simulink model "L7"  (R2023b)
settings: Solver=VariableStepAuto  StartTime=0.0  StopTime=100  MaxStep=0.01  RelTol=1e-3
values from neighbouring files (symbols this model uses):
  Ad = [ 0 1 0 ; 0 0 1 ;  -m0  -m1  -m2 ]    [mL7.m]
  Bd = [ 0 ; 0 ; 1 ]    [mL7.m]
  Cd = [ n0   n1   n2 ]    [mL7.m]
  F = acker (Ad,Bd,poles_mr)    [mL7.m]
  K = 1/pmr_ust    [mL7.m]
  K1 = 0.5    [mL7.m]
  K2 = 0.1    [mL7.m]
  Kg = 1/(K1*K2)    (= 20)    [mL7.m]
  m0 = Wzoh_plant.Denominator{1}(4)    [mL7.m]
  m1 = Wzoh_plant.Denominator{1}(3)    [mL7.m]
  m2 = Wzoh_plant.Denominator{1}(2)    [mL7.m]
  q = 0.2    [mL7.m]
  T1 = 4    [mL7.m]
  T2 = 5    [mL7.m]
  T3 = 1    [mL7.m]
  Ts = 0.1* (T1 + T2 + T3)    (= 1)    [mL7.m]
  Un = 80    [mL7.m]
settings Model: Creator=td  LastModifiedBy=killer
settings SolverCC: AlgebraicLoopSolver=TrustRegion
settings DataIOCC: ReturnWorkspaceOutputs=off
settings DebuggingCC: UnconnectedInputMsg=warning  UnconnectedOutputMsg=warning  UnconnectedLineMsg=warning  ArithmeticOperatorsInVariantConditions=warning
settings ModelReferenceCC: EnableRefExpFcnMdlSchedulingChecks=on
settings SFSimCC: CustomCodeUndefinedFunction=UseInterfaceOnly

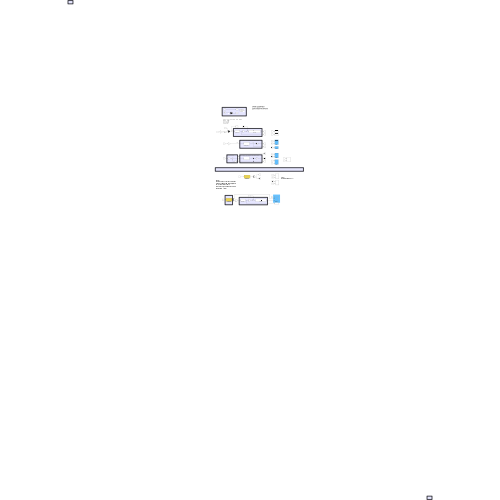
[thumbnail: Simulink's stored preview of the top-level diagram]
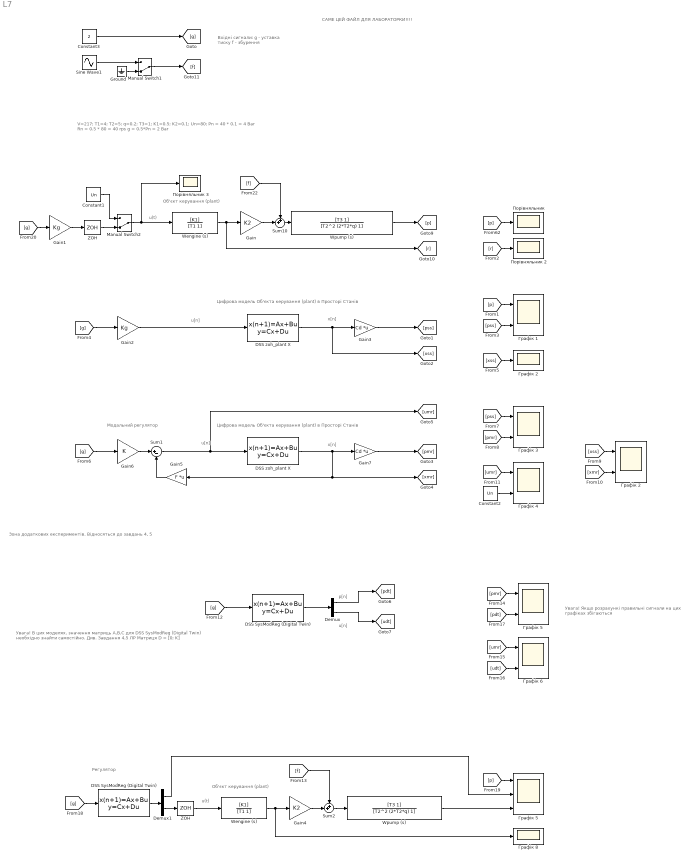
== system L7 ==
  note: Увага!
      | В цих моделях, значення матриць A,B,C для DSS SysModReg (Digital Twin) необхідно знайти самостійно. Див. Завдання 4,5 ЛР
      | Матриця D = [0; K]
  note: Зона додаткових експериментів. Відносяться до завдань 4, 5
  note: Регулятор
  note: Модальний регулятор
  note: x[n]
  note: u(t)
  note: V=217; T1=4; T2=5; q=0.2; T3=1; K1=0.5; K2=0.1; Un=80;
      |
      | Pn = 40 * 0.1 = 4 Bar
      | Rn = 0.5 * 80 = 40 rps
      |
      | g = 0.5*Pn = 2 Bar
  note: Вхідні сигнали:
      |
      | g - уставка тиску
      |
      | f - збурення
  note: САМЕ ЦЕЙ ФАЙЛ
      | ДЛЯ ЛАБОРАТОРКИ!!!!
  note: Об'єкт керування (plant)
  note: Цифрова модель Об'єкта керування (plant) в Просторі Станів
  note: u[n]
  note: Цифрова модель Об'єкта керування (plant) в Просторі Станів
  note: u[n]
  note: x[n]
  note: u(t)
  note: Об'єкт керування (plant)
  note: u[n]
  note: p[n]
  note: Увага!
      | Якщо розрахункі правильні
      | сигнали на цих графіках збігаються
  "  Wpump (s)" : TransferFcn  Numerator=[T3 1]  Denominator=[T2^2 (2*T2*q) 1]
  "  Wpump (s) " : TransferFcn  Numerator=[T3 1]  Denominator=[T2^2 (2*T2*q) 1]
  " DSS SysModReg (Digital Twin)" : DiscreteStateSpace  A=(Ad-Bd*F)  B=Bd*K  C=[Cd; -F]  D=[0; K]  SampleTime=Ts
  " DSS SysModReg (Digital Twin) " : DiscreteStateSpace  A=Ad-Bd*F  B=Bd*K  C=[Cd; -F]  D=[0; K]  SampleTime=Ts
  " DSS zoh_plant X" : DiscreteStateSpace  A="[ 0 1 0 ; 0 0 1 ;  -m0  -m1  -m2 ]"  B=[ 0 ; 0 ; 1 ]  C=eye(3)  D=[0;0;0]  SampleTime=Ts
  " DSS zoh_plant X " : DiscreteStateSpace  A="[ 0 1 0 ; 0 0 1 ;  -m0  -m1  -m2 ]"  B=[ 0 ; 0 ; 1 ]  C=[1 0 0; 0 1 0; 0 0 1]  D=[0;0;0]  SampleTime=Ts
  " ZOH " : ZeroOrderHold  SampleTime=Ts
  " Графік 2" : Scope
  " Графік 5  " : Scope  NumInputPorts=3
  " Порівняльник " : Scope
  " Порівняльник 2" : Scope
  " Порівняльник 3" : Scope
  Constant1 : Constant  Value=Un
  Constant2 : Constant  Value=Un
  Constant3 : Constant  Value=2
  Demux : Demux  Outputs=2
  Demux1 : Demux  Outputs=2
  Gain : Gain  Gain=K2
  Gain1 : Gain  Gain=Kg
  Gain2 : Gain  Gain=Kg
  Gain3 : Gain  Gain=Cd  Multiplication=Matrix(K*u)
  Gain4 : Gain  Gain=K2
  Gain5 : Gain  Gain=F  Multiplication=Matrix(K*u)
  Gain6 : Gain  Gain=K
  Gain7 : Gain  Gain=Cd  Multiplication=Matrix(K*u)
  Ground : Ground
  Manual Switch1 : ManualSwitch  CurrentSetting=0
  Manual Switch2 : ManualSwitch  CurrentSetting=0
  Sine Wave1 : Sin  Amplitude=5  Frequency=0.4  SampleTime=Ts
  Sum1 : Sum  Inputs=|+-
  Sum10 : Sum  Inputs=++|
  Sum2 : Sum  Inputs=++|
  "Wengine (s) " : TransferFcn  Numerator=[K1]  Denominator=[T1 1]
  "Wengine (s)  " : TransferFcn  Numerator=[K1]  Denominator=[T1 1]
  ZOH : ZeroOrderHold  SampleTime=Ts
  Графік {1..6} (6 alike) : Scope  NumInputPorts=2
  Графік 8 : Scope
  wires:
  Sine Wave1/1 -> Manual Switch1/1
  Gain/1 -> Sum10/2
  Sum10/1 -> "  Wpump (s)"/1
  Manual Switch1/1 -> [f]
  "  Wpump (s)"/1 -> [p]
  [f] -> Sum10/1
  Constant3/1 -> [g]
  "Wengine (s) "/1 -> Gain/1, [r]
  [p] -> " Порівняльник "/1
  Manual Switch2/1 -> "Wengine (s) "/1, " Порівняльник 3"/1
  ZOH/1 -> Manual Switch2/2
  Constant1/1 -> Manual Switch2/1
  Ground/1 -> Manual Switch1/2
  [r] -> " Порівняльник 2"/1
  Gain1/1 -> ZOH/1
  [g] -> Gain1/1
  Gain2/1 -> " DSS zoh_plant X "/1
  " DSS zoh_plant X "/1 -> [xss], Gain3/1
  Gain3/1 -> [pss]
  [p] -> Графік 1/1
  [pss] -> Графік 1/2
  [g] -> Gain2/1
  [xss] -> " Графік 2"/1
  " DSS zoh_plant X"/1 -> Gain5/1, [xmr], Gain7/1
  Gain7/1 -> [pmr]
  [g] -> Gain6/1
  Gain6/1 -> Sum1/1
  Sum1/1 -> [umr], " DSS zoh_plant X"/1
  Gain5/1 -> Sum1/2
  [pmr] -> Графік 3/2
  [pss] -> Графік 3/1
  [xss] -> Графік 2/1
  [xmr] -> Графік 2/2
  [umr] -> Графік 4/1
  Constant2/1 -> Графік 4/2
  [g] -> " DSS SysModReg (Digital Twin)"/1
  " DSS SysModReg (Digital Twin)"/1 -> Demux/1
  Demux/1 -> [pdt]
  Demux/2 -> [udt]
  [umr] -> Графік 6/1
  [udt] -> Графік 6/2
  [pdt] -> Графік 5/2
  [pmr] -> Графік 5/1
  "Wengine (s)  "/1 -> Графік 8/1, Gain4/1
  [f] -> Sum2/1
  Gain4/1 -> Sum2/2
  Sum2/1 -> "  Wpump (s) "/1
  [g] -> " DSS SysModReg (Digital Twin) "/1
  " DSS SysModReg (Digital Twin) "/1 -> Demux1/1
  Demux1/2 -> " ZOH "/1
  " ZOH "/1 -> "Wengine (s)  "/1
  [p] -> " Графік 5  "/1
  "  Wpump (s) "/1 -> " Графік 5  "/3
  Demux1/1 -> " Графік 5  "/2
